simulink model "sim_VRPN"  (R2021a)
settings: Solver=FixedStepDiscrete  StartTime=0.0  StopTime=inf  FixedStep=0.002  RelTol=1e-3  EnableMultiTasking=on
libraries: quarc_library x11, simulink_extras x6
settings Model: ExtModeTrigDuration=10000  Creator=glai  LastModifiedBy=glai
settings SolverCC: AlgebraicLoopSolver=TrustRegion  PositivePriorityOrder=on
settings DataIOCC: ReturnWorkspaceOutputs=off
settings DebuggingCC: SFMachineParentedDataDiag=warning  ArithmeticOperatorsInVariantConditions=warning
settings SFSimCC: SimUseLocalCustomCode=off  CustomCodeUndefinedFunction=UseInterfaceOnly
settings RTWCC: Description=QUARC Win64 Target Using Toolchain  SystemTargetFile=quarc_win64.tlc  TemplateMakefile=quarc_default_tmf  RTWUseLocalCustomCode=off  Toolchain=QUARC win64 | nmake (64-bit Windows)  BuildConfiguration=Faster Runs
settings CodeAppCC: StateflowObjectComments=on
settings STFCustomTargetCC: TargetLangStandard=C99 (ISO)  ConcurrentExecutionCompliant=on  SystemTargetFile=quarc_win64.tlc
settings GRTTargetCC: ParMdlRefBuildCompliant=off  CompOptLevelCompliant=off  CombineOutputUpdateFcns=off  MatFileLogging=off  CPPClassGenCompliant=off  GRTInterface=on  ExtMode=on  ExtModeMexFile=quarc_comm
settings ConfigComp: CovMetricSettings=dswe

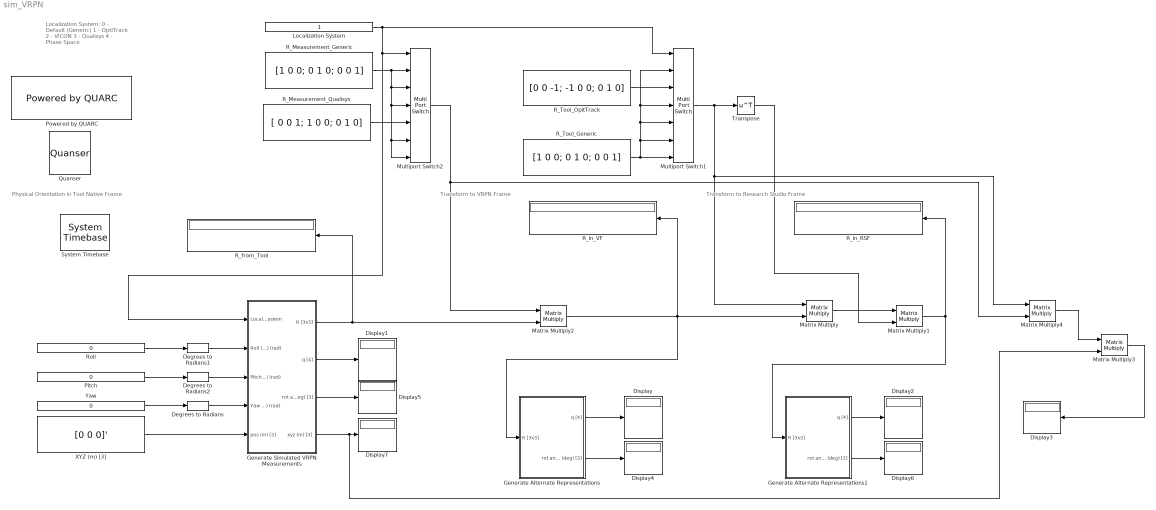
== system sim_VRPN ==
  note: Localization System:
      | 0 - Default (Generic)
      | 1 - OptiTrack
      | 2 - VICON
      | 3 - Qualisys
      | 4 - Phase Space
  note: Transform to Research Studio Frame
  note: Physical Orientation in Tool Native Frame
  note: Transform to VRPN Frame
  Degrees to Radians : simulink_extras/Transformations/Degrees to Radians
  Degrees to Radians1 : simulink_extras/Transformations/Degrees to Radians
  Degrees to Radians2 : simulink_extras/Transformations/Degrees to Radians
  Display{,1..7} (8 alike) : Display
  Generate Alternate Representations : Subsystem
  Generate Alternate Representations1 : Subsystem
  Generate Simulated VRPN Measurements : Subsystem
  Localization System : Constant
  Matrix Multiply{,1..4} (5 alike) : Product  Multiplication=Matrix(*)
  Multiport Switch1 : MultiPortSwitch  DataPortOrder=Zero-based contiguous  Inputs=5  DataPortForDefault=Additional data port  DiagnosticForDefault=Warning  zeroidx=on
  Multiport Switch2 : MultiPortSwitch  DataPortOrder=Zero-based contiguous  Inputs=5  DataPortForDefault=Additional data port  DiagnosticForDefault=Warning  zeroidx=on
  Pitch : Constant  Value=0
  Powered by QUARC : quarc_library/Logos/Powered by QUARC
  Quanser : quarc_library/Logos/Quanser
  R_Measurement_Generic : Constant  Value=[1 0 0; 0 1 0; 0 0 1]  VectorParams1D=off
  R_Measurement_Qualisys : Constant  Value=[ 0 0 1; 1 0 0; 0 1 0]  VectorParams1D=off
  R_Tool_Generic : Constant  Value=[1 0 0; 0 1 0; 0 0 1]  VectorParams1D=off
  R_Tool_OpitTrack : Constant  Value=[0 0 -1; -1 0 0; 0 1 0]  VectorParams1D=off
  R_from_Tool : Display
  R_in_RSF : Display
  R_in_VF : Display
  Roll : Constant  Value=0
  System Timebase : quarc_library/Advanced/Timing/System Timebase  stop_on_overrun=off
      settings: SourceProductName=QUARC Targets
  Transpose : Math  Operator=transpose  SaturateOnIntegerOverflow=on
  XYZ (m) [3] : Constant  Value=[0 0 0]'  VectorParams1D=off
  Yaw : Constant  Value=0
  wires:
  Multiport Switch1/1 -> Matrix Multiply4/1, Matrix Multiply/1, Transpose/1
  Matrix Multiply/1 -> Matrix Multiply1/1
  Matrix Multiply2/1 -> Generate Alternate Representations/1(R [3x3]), Matrix Multiply/2, R_in_VF/1
  Yaw/1 -> Degrees to Radians/1
  Roll/1 -> Degrees to Radians1/1
  Pitch/1 -> Degrees to Radians2/1
  Localization System/1 -> Generate Simulated VRPN Measurements/1(Localization System), Multiport Switch2/1, Multiport Switch1/1
  R_Tool_OpitTrack/1 -> Multiport Switch1/3
  R_Tool_Generic/1 -> Multiport Switch1/5, Multiport Switch1/2, Multiport Switch1/4, Multiport Switch1/6, Multiport Switch1/7
  R_Measurement_Qualisys/1 -> Multiport Switch2/5
  Generate Alternate Representations/2(rot angles (deg) [3]) -> Display4/1
  Matrix Multiply1/1 -> Generate Alternate Representations1/1(R [3x3]), R_in_RSF/1
  R_Measurement_Generic/1 -> Multiport Switch2/3, Multiport Switch2/4, Multiport Switch2/6, Multiport Switch2/7, Multiport Switch2/2
  Generate Alternate Representations/1(q [4]) -> Display/1
  Generate Simulated VRPN Measurements/1(R [3x3]) -> Matrix Multiply2/2, R_from_Tool/1
  Generate Simulated VRPN Measurements/2(q [4]) -> Display1/1
  Generate Simulated VRPN Measurements/3(rot angles (deg) [3]) -> Display5/1
  Generate Alternate Representations1/1(q [4]) -> Display2/1
  Generate Alternate Representations1/2(rot angles (deg) [3]) -> Display6/1
  Degrees to Radians1/1 -> Generate Simulated VRPN Measurements/2(Roll (sideway) (rad))
  Degrees to Radians2/1 -> Generate Simulated VRPN Measurements/3(Pitch (nose up/down) (rad))
  Degrees to Radians/1 -> Generate Simulated VRPN Measurements/4(Yaw (heading) (rad))
  Multiport Switch2/1 -> Matrix Multiply4/2, Matrix Multiply2/1
  Transpose/1 -> Matrix Multiply1/2
  Matrix Multiply3/1 -> Display3/1
  Matrix Multiply4/1 -> Matrix Multiply3/1
  Generate Simulated VRPN Measurements/4(xyz (m) [3]) -> Matrix Multiply3/2, Display7/1
  XYZ (m) [3]/1 -> Generate Simulated VRPN Measurements/5(pos (m) [3])

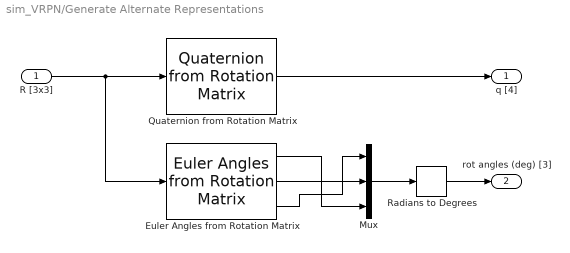
== system sim_VRPN/Generate Alternate Representations ==
  R [3x3] : Inport
  Euler Angles from Rotation Matrix : quarc_library/Math Operations/Matrices/Euler Angles from Rotation Matrix  menu_order=Relative Z-Y-X
      settings: SourceProductName=QUARC Targets
  Mux : Mux  Inputs=3
  Quaternion from Rotation Matrix : quarc_library/Math Operations/Quaternions/Quaternion from Rotation Matrix
      settings: SourceProductName=QUARC Targets
  Radians to Degrees : simulink_extras/Transformations/Radians to Degrees
  q [4] : Outport
  rot angles (deg) [3] : Outport  Port=2
  wires:
  Euler Angles from Rotation Matrix/2 -> Mux/2
  Euler Angles from Rotation Matrix/3 -> Mux/1
  Quaternion from Rotation Matrix/1 -> q [4]/1
  Mux/1 -> Radians to Degrees/1
  Euler Angles from Rotation Matrix/1 -> Mux/3
  R [3x3]/1 -> Euler Angles from Rotation Matrix/1, Quaternion from Rotation Matrix/1
  Radians to Degrees/1 -> rot angles (deg) [3]/1

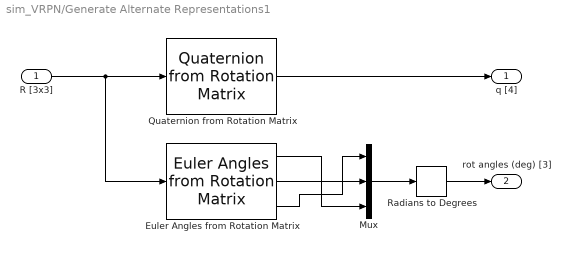
== system sim_VRPN/Generate Alternate Representations1 ==
  R [3x3] : Inport
  Euler Angles from Rotation Matrix : quarc_library/Math Operations/Matrices/Euler Angles from Rotation Matrix  menu_order=Relative Z-Y-X
      settings: SourceProductName=QUARC Targets
  Mux : Mux  Inputs=3
  Quaternion from Rotation Matrix : quarc_library/Math Operations/Quaternions/Quaternion from Rotation Matrix
      settings: SourceProductName=QUARC Targets
  Radians to Degrees : simulink_extras/Transformations/Radians to Degrees
  q [4] : Outport
  rot angles (deg) [3] : Outport  Port=2
  wires:
  Radians to Degrees/1 -> rot angles (deg) [3]/1
  R [3x3]/1 -> Quaternion from Rotation Matrix/1, Euler Angles from Rotation Matrix/1
  Euler Angles from Rotation Matrix/1 -> Mux/3
  Mux/1 -> Radians to Degrees/1
  Quaternion from Rotation Matrix/1 -> q [4]/1
  Euler Angles from Rotation Matrix/3 -> Mux/1
  Euler Angles from Rotation Matrix/2 -> Mux/2

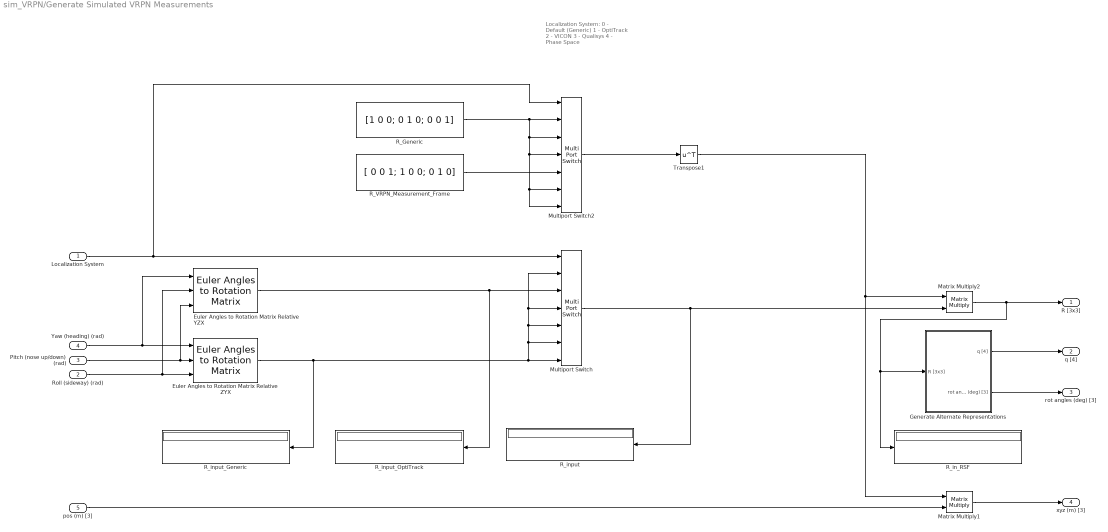
== system sim_VRPN/Generate Simulated VRPN Measurements ==
  note: Localization System:
      | 0 - Default (Generic)
      | 1 - OptiTrack
      | 2 - VICON
      | 3 - Qualisys
      | 4 - Phase Space
  Localization System : Inport
  Roll (sideway) (rad) : Inport  Port=2
  Pitch (nose up/down) (rad) : Inport  Port=3
  Yaw (heading) (rad) : Inport  Port=4
  pos (m) [3] : Inport  Port=5
  Euler Angles to Rotation Matrix Relative YZX : quarc_library/Math Operations/Matrices/Euler Angles to Rotation Matrix  menu_order=Relative Y-Z-X
      settings: SourceProductName=QUARC Targets
  Euler Angles to Rotation Matrix Relative ZYX : quarc_library/Math Operations/Matrices/Euler Angles to Rotation Matrix  menu_order=Relative Z-Y-X
      settings: SourceProductName=QUARC Targets
  Generate Alternate Representations : Subsystem
  Matrix Multiply1 : Product  Multiplication=Matrix(*)
  Matrix Multiply2 : Product  Multiplication=Matrix(*)
  Multiport Switch : MultiPortSwitch  DataPortOrder=Zero-based contiguous  Inputs=5  DataPortForDefault=Additional data port  DiagnosticForDefault=Warning  zeroidx=on
  Multiport Switch2 : MultiPortSwitch  DataPortOrder=Zero-based contiguous  Inputs=5  DataPortForDefault=Additional data port  DiagnosticForDefault=Warning  zeroidx=on
  R_Generic : Constant  Value=[1 0 0; 0 1 0; 0 0 1]  VectorParams1D=off
  R_VRPN_Measurement_Frame : Constant  Value=[ 0 0 1; 1 0 0; 0 1 0]  VectorParams1D=off
  R_in_RSF : Display
  R_input : Display
  R_input_Generic : Display
  R_input_OptiTrack : Display
  Transpose1 : Math  Operator=transpose  SaturateOnIntegerOverflow=on
  R [3x3] : Outport
  q [4] : Outport  Port=2
  rot angles (deg) [3] : Outport  Port=3
  xyz (m) [3] : Outport  Port=4
  wires:
  Localization System/1 -> Multiport Switch2/1, Multiport Switch/1
  Euler Angles to Rotation Matrix Relative YZX/1 -> R_input_OptiTrack/1, Multiport Switch/3
  Euler Angles to Rotation Matrix Relative ZYX/1 -> R_input_Generic/1, Multiport Switch/4, Multiport Switch/2, Multiport Switch/5, Multiport Switch/6, Multiport Switch/7
  Yaw (heading) (rad)/1 -> Euler Angles to Rotation Matrix Relative ZYX/1, Euler Angles to Rotation Matrix Relative YZX/1
  Pitch (nose up/down) (rad)/1 -> Euler Angles to Rotation Matrix Relative YZX/3, Euler Angles to Rotation Matrix Relative ZYX/2
  Roll (sideway) (rad)/1 -> Euler Angles to Rotation Matrix Relative ZYX/3, Euler Angles to Rotation Matrix Relative YZX/2
  Multiport Switch/1 -> R_input/1, Matrix Multiply2/2
  R_VRPN_Measurement_Frame/1 -> Multiport Switch2/5
  Multiport Switch2/1 -> Transpose1/1
  Transpose1/1 -> Matrix Multiply2/1, Matrix Multiply1/1
  Matrix Multiply2/1 -> Generate Alternate Representations/1(R [3x3]), R_in_RSF/1, R [3x3]/1
  Generate Alternate Representations/1(q [4]) -> q [4]/1
  Generate Alternate Representations/2(rot angles (deg) [3]) -> rot angles (deg) [3]/1
  R_Generic/1 -> Multiport Switch2/3, Multiport Switch2/4, Multiport Switch2/7, Multiport Switch2/6, Multiport Switch2/2
  Matrix Multiply1/1 -> xyz (m) [3]/1
  pos (m) [3]/1 -> Matrix Multiply1/2

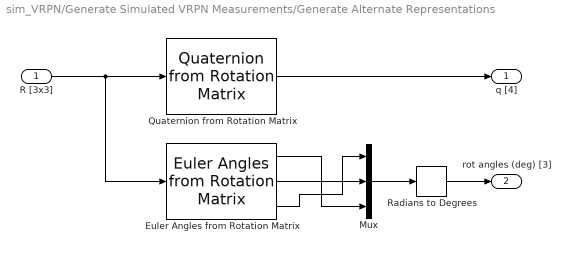
== system sim_VRPN/Generate Simulated VRPN Measurements/Generate Alternate Representations ==
  R [3x3] : Inport
  Euler Angles from Rotation Matrix : quarc_library/Math Operations/Matrices/Euler Angles from Rotation Matrix  menu_order=Relative Z-Y-X
      settings: SourceProductName=QUARC Targets
  Mux : Mux  Inputs=3
  Quaternion from Rotation Matrix : quarc_library/Math Operations/Quaternions/Quaternion from Rotation Matrix
      settings: SourceProductName=QUARC Targets
  Radians to Degrees : simulink_extras/Transformations/Radians to Degrees
  q [4] : Outport
  rot angles (deg) [3] : Outport  Port=2
  wires:
  Euler Angles from Rotation Matrix/2 -> Mux/2
  Euler Angles from Rotation Matrix/3 -> Mux/1
  Quaternion from Rotation Matrix/1 -> q [4]/1
  Mux/1 -> Radians to Degrees/1
  Euler Angles from Rotation Matrix/1 -> Mux/3
  R [3x3]/1 -> Euler Angles from Rotation Matrix/1, Quaternion from Rotation Matrix/1
  Radians to Degrees/1 -> rot angles (deg) [3]/1
